simulink model "test_quad_sim"  (R2025b)
settings: Solver=VariableStepAuto  StartTime=0.0  StopTime=10.0  RelTol=1e-3
PreLoadFcn:
  | init_quadrotor.m
values from neighbouring files (symbols this model uses):
  A = [0 0 0 0 0 0 1 0 0 0 0 0 ... (first row only)    [init_quadrotor.m]
  B = [0 0 0 0 ... (first row only)    [init_quadrotor.m]
  C = eye(12)    [init_quadrotor.m]
  D = zeros(12,4)    [init_quadrotor.m]
  g = params.g    [QuadrotorEOM.m]    (also in QuadrotorPlant.m; init_quadrotor.m = 9.81)
  init_cond = [0; 0; 0 ... (first row only)    [init_quadrotor.m]    (also in temp_main.m = [0; 0; 0;              ang_pert; 0; 0;              0; 0; 0;)
  Kdphi = 5.0    (= 5)    [init_quadrotor.m]
  Kdpsi = 5.0    (= 5)    [init_quadrotor.m]
  Kdtheta = 5.0    (= 5)    [init_quadrotor.m]
  Kdz = 50.0    (= 50)    [init_quadrotor.m]
  Kiphi = 1.0    (= 1)    [init_quadrotor.m]
  Kipsi = 1.0    (= 1)    [init_quadrotor.m]
  Kitheta = 1.0    (= 1)    [init_quadrotor.m]
  Kiz = 40.0    (= 40)    [init_quadrotor.m]
  Kpphi = 10.0    (= 10)    [init_quadrotor.m]
  Kppsi = 10.0    (= 10)    [init_quadrotor.m]
  Kptheta = 10.0    (= 10)    [init_quadrotor.m]
  Kpz = 100.0    (= 100)    [init_quadrotor.m]
  m = 256    [PlotAircraftSim.m]    (also in QuadrotorEOM.m = params.m; QuadrotorPlant.m = params.m; init_quadrotor.m = 5.6)
settings Model: Creator=cooperwark  LastModifiedBy=cooperwark

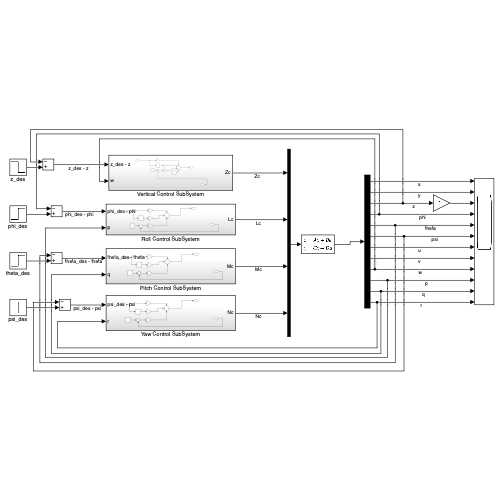
[thumbnail: Simulink's stored preview of the top-level diagram]
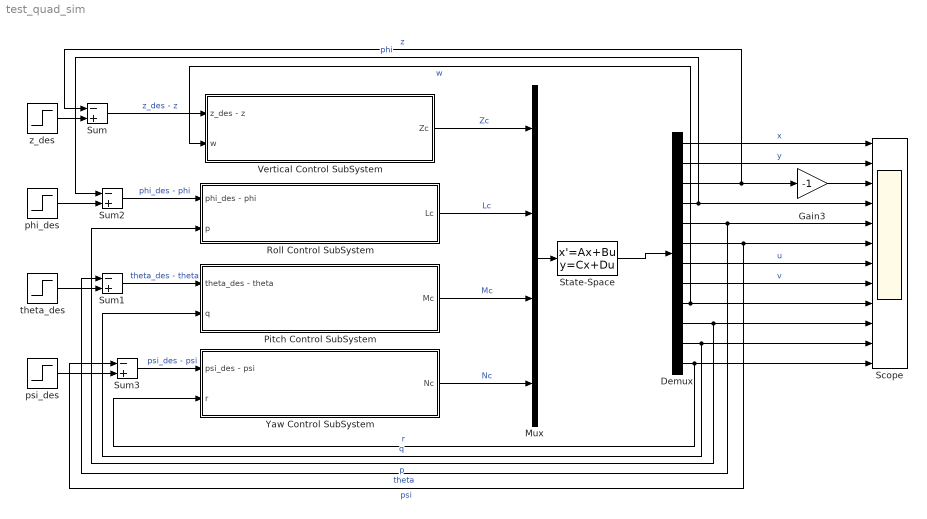
== system test_quad_sim ==
  Demux : Demux  Outputs=12
  Gain3 : Gain  Gain=-1
  Mux : Mux
  Pitch Control SubSystem : Subsystem
  Roll Control SubSystem : Subsystem
  Scope : Scope  NumInputPorts=12
      settings: ActiveDisplayYMinimum=-1  ActiveDisplayYMaximum=1
  State-Space : StateSpace  A=A  B=B  C=C  D=D  InitialCondition=init_cond
  Sum{,1..3} (4 alike) : Sum  Inputs=-+
  Vertical Control SubSystem : Subsystem
  Yaw Control SubSystem : Subsystem
  phi_des : Step  After=0  SampleTime=0
  psi_des : Step  After=0  SampleTime=0
  theta_des : Step  After=0  SampleTime=0
  z_des : Step  After=-2  SampleTime=0
  wires:
  Pitch Control SubSystem/1(Mc) -> Mux/3  "Mc"
  z_des/1 -> Sum/2
  Mux/1 -> State-Space/1
  Demux/3 -> Sum/1, Gain3/1  "z"
  State-Space/1 -> Demux/1
  Sum/1 -> Vertical Control SubSystem/1(z_des - z)  "z_des - z"
  Demux/9 -> Scope/9, Vertical Control SubSystem/2(w)  "w"
  Vertical Control SubSystem/1(Zc) -> Mux/1  "Zc"
  Demux/4 -> Scope/4, Sum2/1  "phi"
  phi_des/1 -> Sum2/2
  Demux/10 -> Roll Control SubSystem/2(p), Scope/10  "p"
  Gain3/1 -> Scope/3
  Demux/1 -> Scope/1  "x"
  Demux/2 -> Scope/2  "y"
  Demux/5 -> Sum1/1, Scope/5  "theta"
  Demux/6 -> Sum3/1, Scope/6  "psi"
  Demux/7 -> Scope/7  "u"
  Demux/8 -> Scope/8  "v"
  Demux/11 -> Pitch Control SubSystem/2(q), Scope/11  "q"
  Demux/12 -> Yaw Control SubSystem/2(r), Scope/12  "r"
  Sum2/1 -> Roll Control SubSystem/1(phi_des - phi)  "phi_des - phi"
  Roll Control SubSystem/1(Lc) -> Mux/2  "Lc"
  Sum1/1 -> Pitch Control SubSystem/1(theta_des - theta)  "theta_des - theta"
  theta_des/1 -> Sum1/2
  Yaw Control SubSystem/1(Nc) -> Mux/4  "Nc"
  Sum3/1 -> Yaw Control SubSystem/1(psi_des - psi)  "psi_des - psi"
  psi_des/1 -> Sum3/2

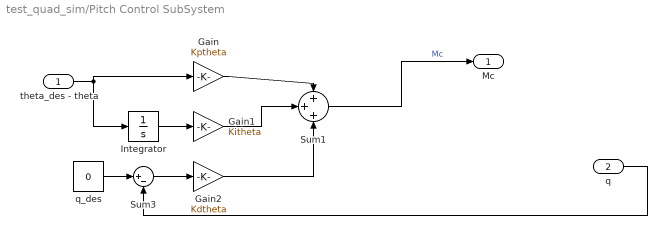
== system test_quad_sim/Pitch Control SubSystem ==
  theta_des - theta : Inport
  q : Inport  Port=2
  Gain : Gain  Gain=Kptheta
  Gain1 : Gain  Gain=Kitheta
  Gain2 : Gain  Gain=Kdtheta
  Integrator : Integrator  LimitOutput=on  UpperSaturationLimit=500  LowerSaturationLimit=-500
  Sum1 : Sum  Inputs=+++
  Sum3 : Sum  Inputs=|+-
  q_des : Constant  Value=0
  Mc : Outport
  wires:
  Sum1/1 -> Mc/1  "Mc"
  theta_des - theta/1 -> Integrator/1, Gain/1
  q/1 -> Sum3/2
  Gain/1 -> Sum1/1
  Sum3/1 -> Gain2/1
  Integrator/1 -> Gain1/1
  q_des/1 -> Sum3/1
  Gain1/1 -> Sum1/2
  Gain2/1 -> Sum1/3

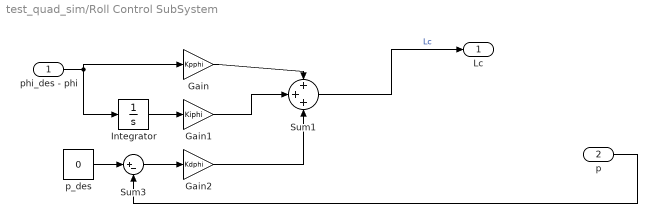
== system test_quad_sim/Roll Control SubSystem ==
  phi_des - phi : Inport
  p : Inport  Port=2
  Gain : Gain  Gain=Kpphi
  Gain1 : Gain  Gain=Kiphi
  Gain2 : Gain  Gain=Kdphi
  Integrator : Integrator  LimitOutput=on  UpperSaturationLimit=500  LowerSaturationLimit=-500
  Sum1 : Sum  Inputs=+++
  Sum3 : Sum  Inputs=|+-
  p_des : Constant  Value=0
  Lc : Outport
  wires:
  Sum1/1 -> Lc/1  "Lc"
  phi_des - phi/1 -> Integrator/1, Gain/1
  p/1 -> Sum3/2
  Gain/1 -> Sum1/1
  Sum3/1 -> Gain2/1
  Integrator/1 -> Gain1/1
  p_des/1 -> Sum3/1
  Gain1/1 -> Sum1/2
  Gain2/1 -> Sum1/3

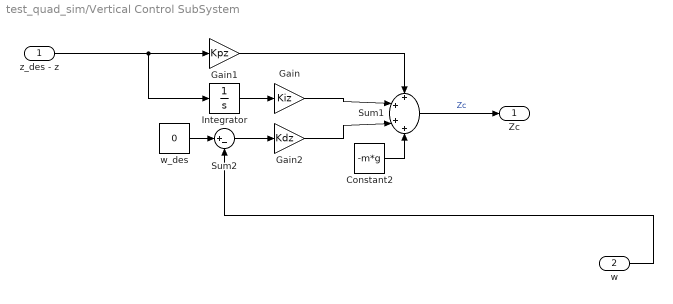
== system test_quad_sim/Vertical Control SubSystem ==
  z_des - z : Inport
  w : Inport  Port=2
  Constant2 : Constant  Value=-m*g
  Gain : Gain  Gain=Kiz
  Gain1 : Gain  Gain=Kpz
  Gain2 : Gain  Gain=Kdz
  Integrator : Integrator  LimitOutput=on  UpperSaturationLimit=500  LowerSaturationLimit=-500
  Sum1 : Sum  Inputs=++++
  Sum2 : Sum  Inputs=|+-
  w_des : Constant  Value=0
  Zc : Outport
  wires:
  w/1 -> Sum2/2
  Constant2/1 -> Sum1/4
  Gain1/1 -> Sum1/1
  Sum1/1 -> Zc/1  "Zc"
  w_des/1 -> Sum2/1
  Integrator/1 -> Gain/1
  z_des - z/1 -> Integrator/1, Gain1/1
  Sum2/1 -> Gain2/1
  Gain2/1 -> Sum1/3
  Gain/1 -> Sum1/2

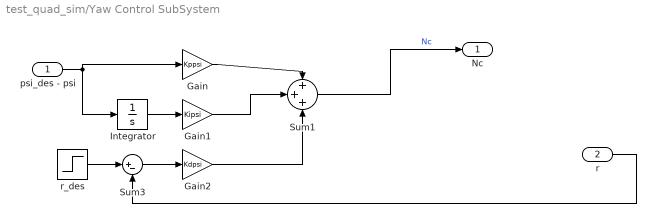
== system test_quad_sim/Yaw Control SubSystem ==
  psi_des - psi : Inport
  r : Inport  Port=2
  Gain : Gain  Gain=Kppsi
  Gain1 : Gain  Gain=Kipsi
  Gain2 : Gain  Gain=Kdpsi
  Integrator : Integrator  LimitOutput=on  UpperSaturationLimit=500  LowerSaturationLimit=-500
  Sum1 : Sum  Inputs=+++
  Sum3 : Sum  Inputs=|+-
  r_des : Step  Time=5  After=0.2  SampleTime=0
  Nc : Outport
  wires:
  Sum1/1 -> Nc/1  "Nc"
  psi_des - psi/1 -> Integrator/1, Gain/1
  r/1 -> Sum3/2
  Gain/1 -> Sum1/1
  Sum3/1 -> Gain2/1
  Integrator/1 -> Gain1/1
  r_des/1 -> Sum3/1
  Gain1/1 -> Sum1/2
  Gain2/1 -> Sum1/3
